simulink model "CRCL"  (R2020b)
settings: Solver=FixedStepDiscrete  StartTime=0.0  StopTime=inf  FixedStep=0.01  RelTol=1e-3  EnableMultiTasking=on
values from neighbouring files (symbols this model uses):
  calibrationDelayTime_s = 2.0    [CRCL_Dictionary.sldd]
  collisionAngleThreshold_deg = 40.0    [CRCL_Dictionary.sldd]
  collisionVarianceThreshold_g2 = 8.0    [CRCL_Dictionary.sldd]
  cpMaxAbortTime_s = 30.0    [CRCL_Dictionary.sldd]
  cpMaxTipOverAngle_deg = 35.0    [CRCL_Dictionary.sldd]
  cpMinEstDistance_m = 50.0    [CRCL_Dictionary.sldd]
  cpMinEstDistanceGnssBased_m = 200.0    [CRCL_Dictionary.sldd]
  cpMinRiddenTime_s = 15.0    [CRCL_Dictionary.sldd]
  cpMinSpeedRiding_kmh = 10.0    [CRCL_Dictionary.sldd]
  cpNumCrankRevolutionThreshold = 5.0    [CRCL_Dictionary.sldd]
  cpSpeedCond2PositiveSpeedChangeTime_s = 5.0    [CRCL_Dictionary.sldd]
  cpSpeedDerivativeThreshold_kmhs = 0.005    [CRCL_Dictionary.sldd]
  cpTimeOutSpeedCond2_s = 15.0    [CRCL_Dictionary.sldd]
  groundHitEnergyThresholdStanding_g2s2 = 0.02    [CRCL_Dictionary.sldd]
  groundHitTipOverAngleThreshold_deg = 40.0    [CRCL_Dictionary.sldd]
  longAccCompForEulerEstFlag = 0.0    [CRCL_Dictionary.sldd]
  minEnergyStrongHit_g2s2 = 0.1    [CRCL_Dictionary.sldd]
  noMotionAccVarianceThresholdSD_g2 = 0.001    [CRCL_Dictionary.sldd]
  ride1minSpeedSlow_kmh = 4.0    [CRCL_Dictionary.sldd]
  ride2minSpeed_kmh = 8.0    [CRCL_Dictionary.sldd]
  rroMaxSpeed_kmh = 5.0    [CRCL_Dictionary.sldd]
  rroMinGyrX_degs = 20.0    [CRCL_Dictionary.sldd]
  rroMonotonyThreshold_degs = -1.0    [CRCL_Dictionary.sldd]
  rroRollIntegrationAngleThreshold_degs = 20.0    [CRCL_Dictionary.sldd]
  rroUniContinuityThreshold_degs = 15.0    [CRCL_Dictionary.sldd]
  scaleFactorVarianceStrongHit = 2.0    [CRCL_Dictionary.sldd]
  sdoMaxAccVarFreeFall_g2 = 0.06    [CRCL_Dictionary.sldd]
  sdoMaxTipOverAngle_deg = 20.0    [CRCL_Dictionary.sldd]
  sdoMinAccVar_g2 = 8.0    [CRCL_Dictionary.sldd]
  sdoMinGyrXYNorm_degs = 720.0    [CRCL_Dictionary.sldd]
  sdoMinGyrXYNormFreeFall_degs = 100.0    [CRCL_Dictionary.sldd]
  sdoMinOrientationChange_deg = 120.0    [CRCL_Dictionary.sldd]
  sdoScaleFactorOrientationChange = 3.0    [CRCL_Dictionary.sldd]
  stepTime_s = 0.01    [CRCL_Dictionary.sldd]
  strongHitSafetyFactor = 2.5    [CRCL_Dictionary.sldd]
  tipOverAccZFiltTreshold_g = 0.7    [CRCL_Dictionary.sldd]
  tipOverAngleThreshold_deg = 50.0    [CRCL_Dictionary.sldd]
  tipOverMinAccZFiltNoseOver_g = 0.3    [CRCL_Dictionary.sldd]
  tipOverRollPitchRelationNoseOver = 1.5    [CRCL_Dictionary.sldd]
undefined symbols (not defined in the file or in its folder): magnitude
libraries: simulink x17
(part 2 of 8)

== system CRCL/Double-Click Button to set current folder ==

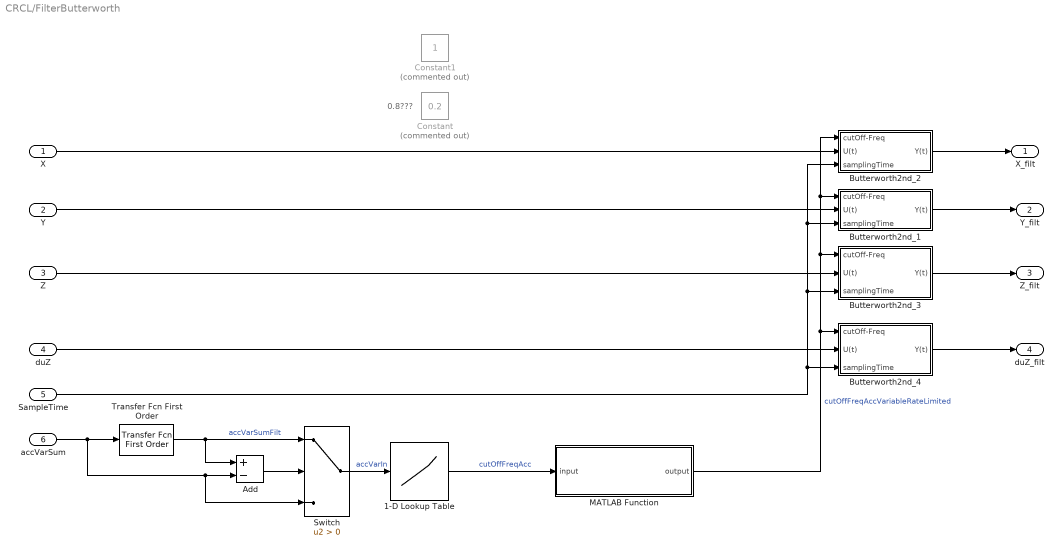
== system CRCL/FilterButterworth ==
  note: 0.8???
  X : Inport
  Y : Inport  Port=2
  Z : Inport  Port=3
  duZ : Inport  Port=4
  SampleTime : Inport  Port=5
  "accVarSum " : Inport  Port=6
  1-D Lookup Table : Lookup_n-D  NumberOfTableDimensions=1  BreakpointsForDimension1=[0 0.0005 0.005 0.01 0.1 50]  Table=[10 10 1 0.5 0.2 0.2]  InternalRulePriority=Speed  RndMeth=Simplest  InputSameDT=on
  Add : Sum  Inputs=+-
  Butterworth2nd_1 : Subsystem
  Butterworth2nd_2 : Subsystem
  Butterworth2nd_3 : Subsystem
  Butterworth2nd_4 : Subsystem
  Constant : Constant  Commented=on  Value=0.2  OutDataTypeStr=single
  Constant1 : Constant  Commented=on
  MATLAB Function : MATLAB Function  TreatAsAtomicUnit=on
  Switch : Switch  Criteria=u2 > Threshold
  Transfer Fcn First Order : simulink/Discrete/Transfer Fcn First Order  PoleZ=0.92  ICPrevOutput=0.0  DoSatur=off
  X_filt : Outport  VectorParamsAs1DForOutWhenUnconnected=off
  Y_filt : Outport  Port=2  VectorParamsAs1DForOutWhenUnconnected=off
  Z_filt : Outport  Port=3  VectorParamsAs1DForOutWhenUnconnected=off
  duZ_filt : Outport  Port=4  VectorParamsAs1DForOutWhenUnconnected=off
  wires:
  Butterworth2nd_2/1(Y(t)) -> X_filt/1
  Butterworth2nd_1/1(Y(t)) -> Y_filt/1
  Butterworth2nd_3/1(Y(t)) -> Z_filt/1
  Z/1 -> Butterworth2nd_3/2(U(t))
  Y/1 -> Butterworth2nd_1/2(U(t))
  X/1 -> Butterworth2nd_2/2(U(t))
  "accVarSum "/1 -> Switch/3, Add/2, Transfer Fcn First Order/1
  Add/1 -> Switch/2
  Transfer Fcn First Order/1 -> Add/1, Switch/1  "accVarSumFilt"
  Switch/1 -> 1-D Lookup Table/1  "accVarIn"
  1-D Lookup Table/1 -> MATLAB Function/1(input)  "cutOffFreqAcc"
  MATLAB Function/1(output) -> Butterworth2nd_4/1(cutOff-Freq), Butterworth2nd_2/1(cutOff-Freq), Butterworth2nd_1/1(cutOff-Freq), Butterworth2nd_3/1(cutOff-Freq)  "cutOffFreqAccVariableRateLimited"
  duZ/1 -> Butterworth2nd_4/2(U(t))
  Butterworth2nd_4/1(Y(t)) -> duZ_filt/1
  SampleTime/1 -> Butterworth2nd_4/3(samplingTime), Butterworth2nd_1/3(samplingTime), Butterworth2nd_2/3(samplingTime), Butterworth2nd_3/3(samplingTime)

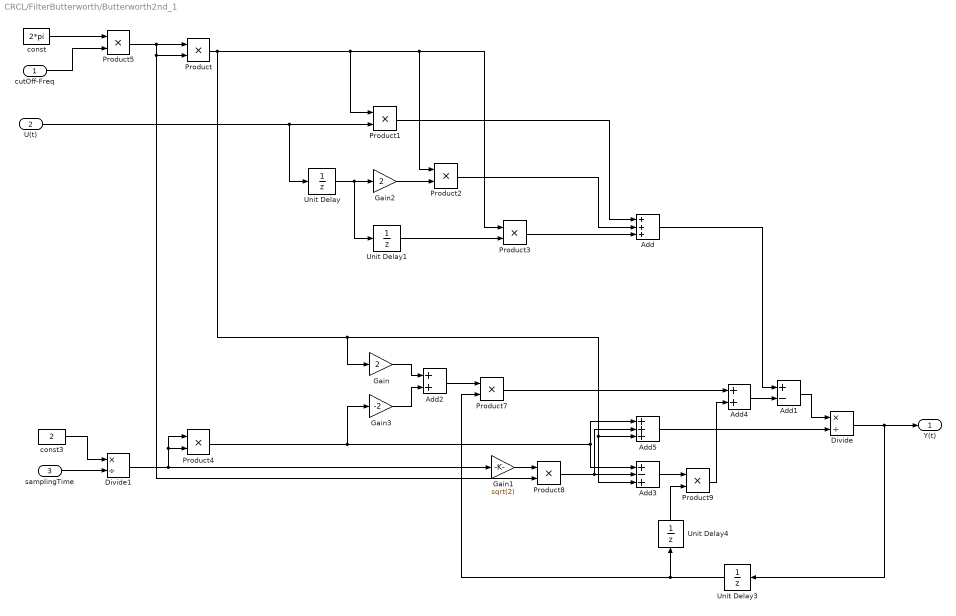
== system CRCL/FilterButterworth/Butterworth2nd_1 ==
  cutOff-Freq : Inport
  U(t) : Inport  Port=2
  samplingTime : Inport  Port=3
  Add : Sum  Inputs=+++
  Add1 : Sum  Inputs=+-
  Add2 : Sum
  Add3 : Sum  Inputs=+-+
  Add4 : Sum
  Add5 : Sum  Inputs=+++
  Divide : Product  Inputs=*/
  Divide1 : Product  Inputs=*/
  Gain : Gain  Gain=2
  Gain1 : Gain  Gain=sqrt(2)
  Gain2 : Gain  Gain=2
  Gain3 : Gain  Gain=-2
  Product{,1..5,7..9} (9 alike) : Product  RndMeth=Zero
  Unit Delay{,1,3..4} (4 alike) : UnitDelay  SampleTime=-1  HasFrameUpgradeWarning=on
  const : Constant  Value=2*pi  OutDataTypeStr=single
  const3 : Constant  Value=2  OutDataTypeStr=single
  Y(t) : Outport  VectorParamsAs1DForOutWhenUnconnected=off
  wires:
  U(t)/1 -> Product1/2, Unit Delay/1
  Product/1 -> Product1/1, Product3/1, Product2/1, Gain/1, Add3/3, Add5/3
  Unit Delay/1 -> Unit Delay1/1, Gain2/1
  Unit Delay1/1 -> Product3/2
  Product1/1 -> Add/1
  Product2/1 -> Add/2
  Product3/1 -> Add/3
  Add/1 -> Add1/1
  Divide/1 -> Unit Delay3/1, Y(t)/1
  Product4/1 -> Add3/1, Add5/1, Gain3/1
  Gain/1 -> Add2/1
  Unit Delay3/1 -> Product7/2, Unit Delay4/1
  Add2/1 -> Product7/1
  Gain1/1 -> Product8/1
  Product8/1 -> Add3/2, Add5/2
  Unit Delay4/1 -> Product9/2
  Add3/1 -> Product9/1
  Product9/1 -> Add4/2
  Product7/1 -> Add4/1
  Add4/1 -> Add1/2
  Add1/1 -> Divide/1
  Add5/1 -> Divide/2
  Gain2/1 -> Product2/2
  Gain3/1 -> Add2/2
  Product5/1 -> Product/1, Product/2, Product8/2
  const/1 -> Product5/1
  cutOff-Freq/1 -> Product5/2
  const3/1 -> Divide1/1
  samplingTime/1 -> Divide1/2
  Divide1/1 -> Gain1/1, Product4/2, Product4/1

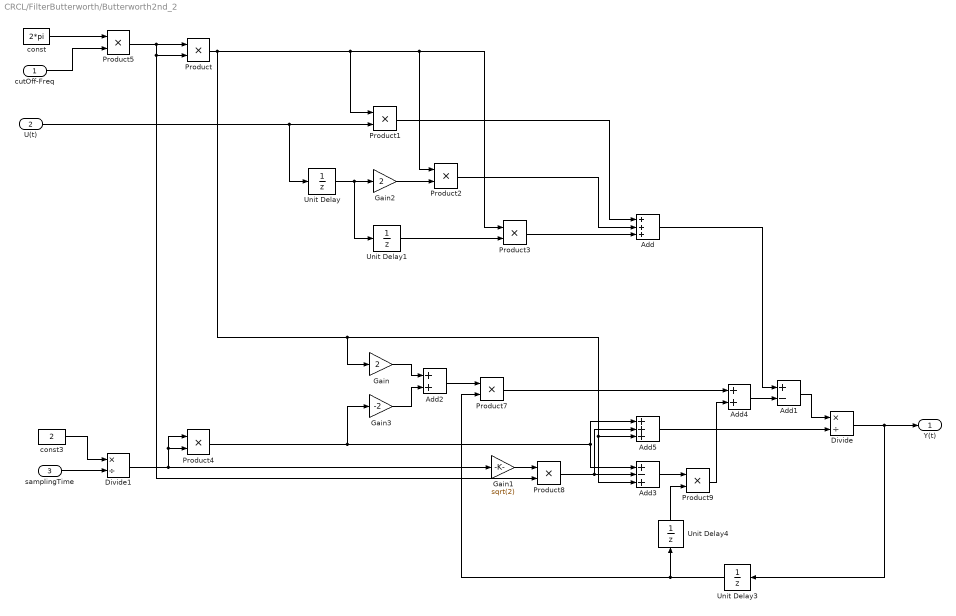
== system CRCL/FilterButterworth/Butterworth2nd_2 ==
  cutOff-Freq : Inport
  U(t) : Inport  Port=2
  samplingTime : Inport  Port=3
  Add : Sum  Inputs=+++
  Add1 : Sum  Inputs=+-
  Add2 : Sum
  Add3 : Sum  Inputs=+-+
  Add4 : Sum
  Add5 : Sum  Inputs=+++
  Divide : Product  Inputs=*/
  Divide1 : Product  Inputs=*/
  Gain : Gain  Gain=2
  Gain1 : Gain  Gain=sqrt(2)
  Gain2 : Gain  Gain=2
  Gain3 : Gain  Gain=-2
  Product{,1..5,7..9} (9 alike) : Product  RndMeth=Zero
  Unit Delay{,1,3..4} (4 alike) : UnitDelay  SampleTime=-1  HasFrameUpgradeWarning=on
  const : Constant  Value=2*pi  OutDataTypeStr=single
  const3 : Constant  Value=2  OutDataTypeStr=single
  Y(t) : Outport  VectorParamsAs1DForOutWhenUnconnected=off
  wires:
  Divide1/1 -> Product4/1, Product4/2, Gain1/1
  samplingTime/1 -> Divide1/2
  const3/1 -> Divide1/1
  cutOff-Freq/1 -> Product5/2
  const/1 -> Product5/1
  Product5/1 -> Product8/2, Product/2, Product/1
  Gain3/1 -> Add2/2
  Gain2/1 -> Product2/2
  Add5/1 -> Divide/2
  Add1/1 -> Divide/1
  Add4/1 -> Add1/2
  Product7/1 -> Add4/1
  Product9/1 -> Add4/2
  Add3/1 -> Product9/1
  Unit Delay4/1 -> Product9/2
  Product8/1 -> Add5/2, Add3/2
  Gain1/1 -> Product8/1
  Add2/1 -> Product7/1
  Unit Delay3/1 -> Unit Delay4/1, Product7/2
  Gain/1 -> Add2/1
  Product4/1 -> Gain3/1, Add5/1, Add3/1
  Divide/1 -> Y(t)/1, Unit Delay3/1
  Add/1 -> Add1/1
  Product3/1 -> Add/3
  Product2/1 -> Add/2
  Product1/1 -> Add/1
  Unit Delay1/1 -> Product3/2
  Unit Delay/1 -> Gain2/1, Unit Delay1/1
  Product/1 -> Add5/3, Add3/3, Gain/1, Product2/1, Product3/1, Product1/1
  U(t)/1 -> Unit Delay/1, Product1/2

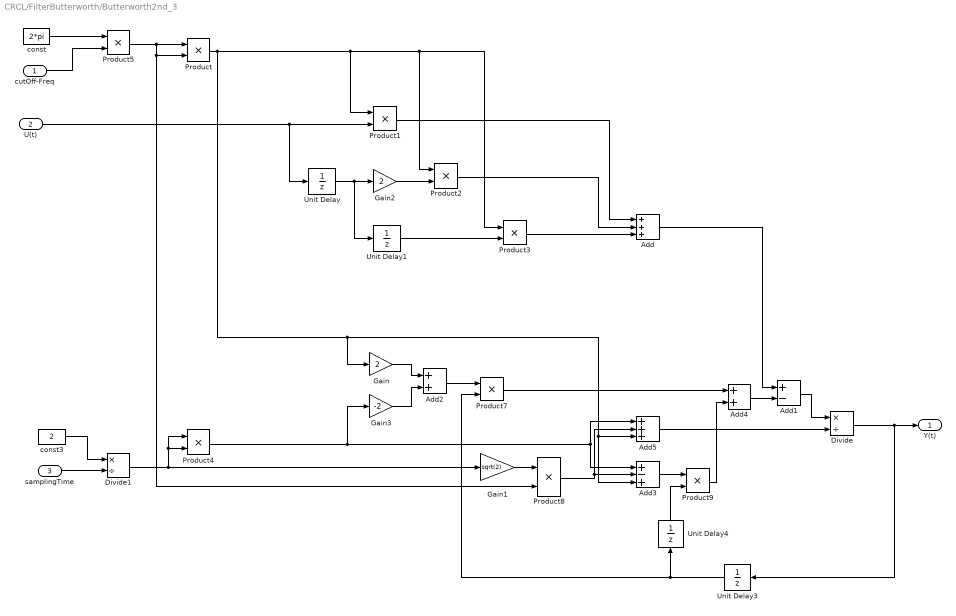
== system CRCL/FilterButterworth/Butterworth2nd_3 ==
  cutOff-Freq : Inport
  U(t) : Inport  Port=2
  samplingTime : Inport  Port=3
  Add : Sum  Inputs=+++
  Add1 : Sum  Inputs=+-
  Add2 : Sum
  Add3 : Sum  Inputs=+-+
  Add4 : Sum
  Add5 : Sum  Inputs=+++
  Divide : Product  Inputs=*/
  Divide1 : Product  Inputs=*/
  Gain : Gain  Gain=2
  Gain1 : Gain  Gain=sqrt(2)
  Gain2 : Gain  Gain=2
  Gain3 : Gain  Gain=-2
  Product{,1..5,7..9} (9 alike) : Product  RndMeth=Zero
  Unit Delay{,1,3..4} (4 alike) : UnitDelay  SampleTime=-1  HasFrameUpgradeWarning=on
  const : Constant  Value=2*pi  OutDataTypeStr=single
  const3 : Constant  Value=2  OutDataTypeStr=single
  Y(t) : Outport  VectorParamsAs1DForOutWhenUnconnected=off
  wires:
  Divide1/1 -> Product4/1, Product4/2, Gain1/1
  samplingTime/1 -> Divide1/2
  const3/1 -> Divide1/1
  cutOff-Freq/1 -> Product5/2
  const/1 -> Product5/1
  Product5/1 -> Product8/2, Product/2, Product/1
  Gain3/1 -> Add2/2
  Gain2/1 -> Product2/2
  Add5/1 -> Divide/2
  Add1/1 -> Divide/1
  Add4/1 -> Add1/2
  Product7/1 -> Add4/1
  Product9/1 -> Add4/2
  Add3/1 -> Product9/1
  Unit Delay4/1 -> Product9/2
  Product8/1 -> Add5/2, Add3/2
  Gain1/1 -> Product8/1
  Add2/1 -> Product7/1
  Unit Delay3/1 -> Unit Delay4/1, Product7/2
  Gain/1 -> Add2/1
  Product4/1 -> Gain3/1, Add5/1, Add3/1
  Add/1 -> Add1/1
  Product3/1 -> Add/3
  Product2/1 -> Add/2
  Product1/1 -> Add/1
  Unit Delay1/1 -> Product3/2
  Unit Delay/1 -> Gain2/1, Unit Delay1/1
  Product/1 -> Add5/3, Add3/3, Gain/1, Product2/1, Product3/1, Product1/1
  U(t)/1 -> Unit Delay/1, Product1/2
  Divide/1 -> Unit Delay3/1, Y(t)/1

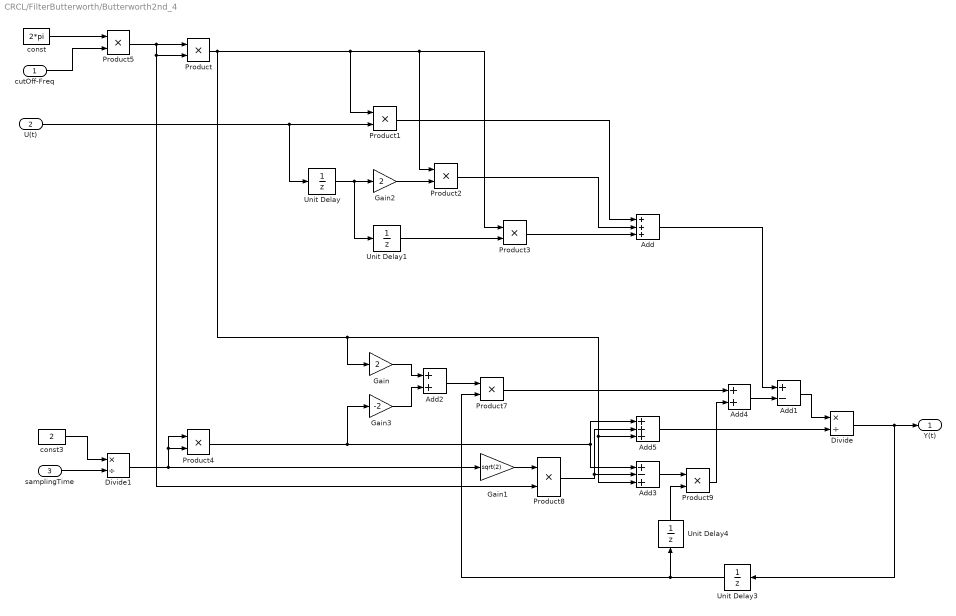
== system CRCL/FilterButterworth/Butterworth2nd_4 ==
  cutOff-Freq : Inport
  U(t) : Inport  Port=2
  samplingTime : Inport  Port=3
  Add : Sum  Inputs=+++
  Add1 : Sum  Inputs=+-
  Add2 : Sum
  Add3 : Sum  Inputs=+-+
  Add4 : Sum
  Add5 : Sum  Inputs=+++
  Divide : Product  Inputs=*/
  Divide1 : Product  Inputs=*/
  Gain : Gain  Gain=2
  Gain1 : Gain  Gain=sqrt(2)
  Gain2 : Gain  Gain=2
  Gain3 : Gain  Gain=-2
  Product{,1..5,7..9} (9 alike) : Product  RndMeth=Zero
  Unit Delay{,1,3..4} (4 alike) : UnitDelay  SampleTime=-1  HasFrameUpgradeWarning=on
  const : Constant  Value=2*pi  OutDataTypeStr=single
  const3 : Constant  Value=2  OutDataTypeStr=single
  Y(t) : Outport  VectorParamsAs1DForOutWhenUnconnected=off
  wires:
  Divide/1 -> Y(t)/1, Unit Delay3/1
  U(t)/1 -> Product1/2, Unit Delay/1
  Product/1 -> Product1/1, Product3/1, Product2/1, Gain/1, Add3/3, Add5/3
  Unit Delay/1 -> Unit Delay1/1, Gain2/1
  Unit Delay1/1 -> Product3/2
  Product1/1 -> Add/1
  Product2/1 -> Add/2
  Product3/1 -> Add/3
  Add/1 -> Add1/1
  Product4/1 -> Add3/1, Add5/1, Gain3/1
  Gain/1 -> Add2/1
  Unit Delay3/1 -> Product7/2, Unit Delay4/1
  Add2/1 -> Product7/1
  Gain1/1 -> Product8/1
  Product8/1 -> Add3/2, Add5/2
  Unit Delay4/1 -> Product9/2
  Add3/1 -> Product9/1
  Product9/1 -> Add4/2
  Product7/1 -> Add4/1
  Add4/1 -> Add1/2
  Add1/1 -> Divide/1
  Add5/1 -> Divide/2
  Gain2/1 -> Product2/2
  Gain3/1 -> Add2/2
  Product5/1 -> Product/1, Product/2, Product8/2
  const/1 -> Product5/1
  cutOff-Freq/1 -> Product5/2
  const3/1 -> Divide1/1
  samplingTime/1 -> Divide1/2
  Divide1/1 -> Gain1/1, Product4/2, Product4/1

== matlab function CRCL/Madgwick IMU MATLAB Function1 ==
  data: AccelerometerX input; AccelerometerY input; AccelerometerZ input; gyrBfX input; gyrBfY input; gyrBfZ input; Beta input; eulerPitch output; eulerRoll output; eulerYaw output; BetaIntern output; SD_fire input; SecondCalibrationDonePeriod input; HD_GroundHit input; HD_CollisionHit input; GyroBiasX output; GyroBiasY output; GyroBiasZ output; SecondCalibrationDone input; curVarSum input
function [eulerPitch, eulerRoll, eulerYaw,...
    BetaIntern, GyroBiasX, GyroBiasY, GyroBiasZ] =  fcn(AccelerometerX, AccelerometerY, AccelerometerZ, ...
    gyrBfX, gyrBfY, gyrBfZ, Beta, SD_fire, SecondCalibrationDonePeriod,...
    HD_GroundHit, HD_CollisionHit, SecondCalibrationDone, curVarSum)

    % calculate centrifugal Acc
    % centrifugalAcc = cross([gyrBfX * pi / 180 ; gyrBfY * pi / 180 ; gyrBfZ * pi / 180],[speed_kmh/3.6; 0; 0]);
    % 
    % centrifualAccX_g = centrifugalAcc(1) / 9.81;
    % centrifualAccY_g = centrifugalAcc(2) / 9.81;
    % centrifualAccZ_g = centrifugalAcc(3) / 9.81;
    % 
    % Accelerometer = [AccelerometerFilteredY + centrifualAccY_g; AccelerometerStrongFilteredX + centrifualAccX_g;...
    %    AccelerometerStrongFilteredZ + centrifualAccZ_g];

%     Accelerometer = [AccelerometerY; AccelerometerX;...
%          AccelerometerZ];
     
    Accelerometer = single([AccelerometerX; AccelerometerY;...
         AccelerometerZ]);
     
     %check Data: if Accelerometer is all zero, Madgwick returns NaN
    if ~any(Accelerometer) 
        Accelerometer = single([0.05; 0.05; 1]);
    end
%     Gyroscope = [gyrBfY; gyrBfX; gyrBfZ];
    Gyroscope = [gyrBfX; gyrBfY; gyrBfZ];

    persistent SamplePeriod Quaternion Step GyroBiasEst Theta gyroBiasFlag

    %% declaration only during first run!

    if isempty(SamplePeriod)
            SamplePeriod = 1/100;
            Quaternion=Start(Accelerometer);
            GyroBiasEst=[0 0 0];
            Theta = 0.000002;
            gyroBiasFlag = 0;
    end

    if SD_fire && (HD_GroundHit == 1 || HD_CollisionHit == 1)
        BetaIntern =  200 * Beta;
    elseif SD_fire == 1 || SecondCalibrationDonePeriod == 1  
        BetaIntern =  100 * Beta;
%     elseif SecondCalibrationDone == 1 && curVarSum <= 0.015
%         BetaIntern =  25 * Beta;
    else
        BetaIntern =  Beta;
    end
    
    q =  Quaternion; % short name local variable for readability, Jan: Quaternion represents Orientation
    Gyroscope = Gyroscope *(pi/180);

    %Centrifugal_acc = cross(Gyroscope, [Speed 0  0])/9.81;      %speed in m/s
    %Accelerometer =  Accelerometer - Centrifugal_acc';
    
	% Gradient decent algorithm corrective Step
            F = [2*(q(2)*q(4) - q(1)*q(3)) - Accelerometer(1)
                2*(q(1)*q(2) + q(3)*q(4))  - Accelerometer(2)
                2*(0.5 - q(2)^2 - q(3)^2)  - Accelerometer(3)];
            J = [-2*q(3),	2*q(4),    -2*q(1),	2*q(2)
                2*q(2),     2*q(1),     2*q(4),	2*q(3)
                0,         -4*q(2),    -4*q(3),	0    ];
	Step = (J'*F);
	Step = Step / norm(Step);	% normalise Step magnitude
    
    if gyroBiasFlag == 1 || SecondCalibrationDonePeriod == 1
        gyroBiasFlag = 1;
        So = 2 * quaternProd(quaternConj(q), (Step / norm(Step))');
        GyroBiasEst = GyroBiasEst + Theta .* So(2:end); 
    end

    
% 	gravity = [2*(q(2)*q(4) - q(1)*q(3))
% 			2*(q(1)*q(2) + q(3)*q(4))
% 			2*(0.5 - q(2)^2 - q(3)^2)];

    % 		So = 2 * quaternProd(quaternConj(q), (Step / norm(Step))');
    % 		qDot = 0.5 * quaternProd(q, [0 Gyroscope(1)- GyroBias(1) Gyroscope(2)- GyroBias(2) Gyroscope(3)- GyroBias(3)]) - BetaIntern * Step';
    qDot = 0.5 * quaternProd(q, [0 Gyroscope(1)-GyroBiasEst(1) Gyroscope(2)-GyroBiasEst(2) Gyroscope(3)-GyroBiasEst(3)]) - BetaIntern * Step';

    % Integrate to yield quaternion
    q = q + qDot *  SamplePeriod;
    Quaternion = q / norm(q); % normalise quaternion
    euler = quatern2euler(quaternConj(Quaternion)) * (180/pi);	% use conjugate for sensor frame relative to Earth and convert to degrees.
    %euler = unwrap(euler,180);
    eulerRoll = euler(1);
    eulerPitch = euler(2);
    eulerYaw = euler(3);
    
    GyroBiasX = GyroBiasEst(1)*180/pi;
    GyroBiasY = GyroBiasEst(2)*180/pi;
    GyroBiasZ = GyroBiasEst(3)*180/pi;
    
end

 function [Quat] = Start(Accelerometer)
    stepper=single([1 1 1 1]');
    Quat=single([1 0 0 0]);
    while norm(stepper) >= 1e-2
        [Quat, stepper]= Update(Accelerometer, single([0 0 0]) , Quat(1,1:4),stepper(1:4));
    end            
 end

function [Quat, stepper] = Update(Accelerometer, Gyroscope, Quat, stepper)

persistent SamplePeriod Quaternion GyroBias Theta Step
%% declaration only during first run!

if isempty(SamplePeriod)
        SamplePeriod = single(1/100);
        Quaternion = single([1 0 0 0]);     % output quaternion describing the Earth relative to the sensor
%         GyroBias = [-1 1 0]*pi/180;
        GyroBias = single([0 0 0]);        
        Theta = single(0.00001);
        Step = single([0 0 0 0]');
     
               
end
% 	euler=zeros(1,3);
	q =  Quaternion; % short name local variable for readability, Jan: Quaternion represents Orientation
           
	BetaIntern = 0.9;
	
	Gyroscope=Gyroscope* (pi/180);
	
	% Normalise accelerometer measurement
	Accelerometer = Accelerometer / norm(Accelerometer);	% normalise magnitude
	% Gradient decent algorithm corrective Step
            F = [2*(q(2)*q(4) - q(1)*q(3)) - Accelerometer(1)
                2*(q(1)*q(2) + q(3)*q(4))  - Accelerometer(2)
                2*(0.5 - q(2)^2 - q(3)^2)  - Accelerometer(3)];
            J = [-2*q(3),	2*q(4),    -2*q(1),	2*q(2)
                2*q(2),     2*q(1),     2*q(4),	2*q(3)
                0,         -4*q(2),    -4*q(3),	0    ];
	Step = (J'*F);
	stepper = Step;
	Step = Step / norm(Step);	% normalise Step magnitude
	
	% Compute rate of change of quaternion
	
	gravity = [2*(q(2)*q(4) - q(1)*q(3))
			2*(q(1)*q(2) + q(3)*q(4))
			2*(0.5 - q(2)^2 - q(3)^2)];

		So = 2 * quaternProd(quaternConj(q), (Step / norm(Step))');
		%GyroBias =  GyroBias +  Theta .* So(2:end);  
		%qDot = 0.5 * quaternProd(q, [0 Gyroscope(1)- GyroBias(1) Gyroscope(2)- GyroBias(2) Gyroscope(3)- GyroBias(3)]) -  Beta * Step';
		qDot = 0.5 * quaternProd(q, [0 Gyroscope(1)- GyroBias(1) Gyroscope(2)- GyroBias(2) Gyroscope(3)- GyroBias(3)]) - BetaIntern * Step';
	
	% Integrate to yield quaternion
	q = q + qDot *  SamplePeriod;
	Quaternion = q / norm(q); % normalise quaternion
	Quat=Quaternion;
%              euler = quatern2euler(quaternConj(Quaternion)) * (180/pi);	% use conjugate for sensor frame relative to Earth and convert to degrees.
%              euler = unwrap(euler,180);

end

function euler = quatern2euler(q)
%QUATERN2EULER Converts a quaternion orientation to ZYX Euler angles
%
%   q = quatern2euler(q)
%
%   Converts a quaternion orientation to ZYX Euler angles where phi is a
%   rotation around X, theta around Y and psi around Z.
%
%   For more information see:
%   http://www.x-io.co.uk/node/8#quaternions
%
%	Date          Author          Notes
%	27/09/2011    SOH Madgwick    Initial release
% R = zeros(3,3,1);
%     R(1,1,:) = 2.*q(:,1).^2-1+2.*q(:,2).^2;
%     R(2,1,:) = 2.*(q(:,2).*q(:,3)-q(:,1).*q(:,4));
%     R(3,1,:) = 2.*(q(:,2).*q(:,4)+q(:,1).*q(:,3));
%     R(3,2,:) = 2.*(q(:,3).*q(:,4)-q(:,1).*q(:,2));
%     R(3,3,:) = 2.*q(:,1).^2-1+2.*q(:,4).^2;
% 
%     phi = atan2(R(3,2,:), R(3,3,:) );
%     theta = -atan(R(3,1,:) ./ sqrt(1-R(3,1,:).^2) );
%     psi = atan2(R(2,1,:), R(1,1,:) );
% 
%     euler = [phi(1,:)' theta(1,:)' psi(1,:)'];
    
    R = zeros(3,3);
    R(1,1) = 2.*q(1).^2-1+2.*q(2).^2;
    R(2,1) = 2.*(q(2).*q(3)-q(1).*q(4));
    R(3,1) = 2.*(q(2).*q(4)+q(1).*q(3));
    R(3,2) = 2.*(q(3).*q(4)-q(1).*q(2));
    R(3,3) = 2.*q(1).^2-1+2.*q(4).^2;

    phi = atan2(R(3,2), R(3,3));
    theta = -atan(R(3,1) ./ sqrt(1-R(3,1).^2) );
    psi = atan2(R(2,1), R(1,1) );

    euler = [phi theta psi];
end

function qConj = quaternConj(q)
%QUATERN2ROTMAT Converts a quaternion to its conjugate
%
%   qConj = quaternConj(q)
%
%   Converts a quaternion to its conjugate.
%
%   For more information see:
%   http://www.x-io.co.uk/node/8#quaternions
%
%	Date          Author          Notes
%	27/09/2011    SOH Madgwick    Initial release

    qConj = [q(:,1) -q(:,2) -q(:,3) -q(:,4)];
end


function ab = quaternProd(a, b)
%QUATERNPROD Calculates the quaternion product
%
%   ab = quaternProd(a, b)
%
%   Calculates the quaternion product of quaternion a and b.
%
%   For more information see:
%   http://www.x-io.co.uk/node/8#quaternions
%
%	Date          Author          Notes
%	27/09/2011    SOH Madgwick    Initial release
%     ab = zeros(1,4);
%     ab(:,1) = a(:,1).*b(:,1)-a(:,2).*b(:,2)-a(:,3).*b(:,3)-a(:,4).*b(:,4);
%     ab(:,2) = a(:,1).*b(:,2)+a(:,2).*b(:,1)+a(:,3).*b(:,4)-a(:,4).*b(:,3);
%     ab(:,3) = a(:,1).*b(:,3)-a(:,2).*b(:,4)+a(:,3).*b(:,1)+a(:,4).*b(:,2);
%     ab(:,4) = a(:,1).*b(:,4)+a(:,2).*b(:,3)-a(:,3).*b(:,2)+a(:,4).*b(:,1);
%     
        ab = zeros(1,4);
    ab(1,1) = a(1,1).*b(1,1)-a(1,2).*b(1,2)-a(1,3).*b(1,3)-a(1,4).*b(1,4);
    ab(1,2) = a(1,1).*b(1,2)+a(1,2).*b(1,1)+a(1,3).*b(1,4)-a(1,4).*b(1,3);
    ab(1,3) = a(1,1).*b(1,3)-a(1,2).*b(1,4)+a(1,3).*b(1,1)+a(1,4).*b(1,2);
    ab(1,4) = a(1,1).*b(1,4)+a(1,2).*b(1,3)-a(1,3).*b(1,2)+a(1,4).*b(1,1);
end

function q = angle2quatern( r1, r2, r3 )


angles = [r1 r2 r3];

cang = cos( angles/2 );
sang = sin( angles/2 );

        q = [ cang(1).*cang(2).*cang(3) + sang(1).*sang(2).*sang(3), ...
            cang(1).*cang(2).*sang(3) - sang(1).*sang(2).*cang(3), ...
            cang(1).*sang(2).*cang(3) + sang(1).*cang(2).*sang(3), ...
            sang(1).*cang(2).*cang(3) - cang(1).*sang(2).*sang(3)];
end

== stateflow chart CRCL/StandDetection_SD ==
  state StandDetectionWithoutSpeed [parallel]
    settings: executionOrder=1
    state Init
      en:
      SD_StandFire = int16(1);
    note: only IMU based, no Speed
    state waitState
    state CheckVarianceStillRiding
    state Riding
    state Standing
    state CheckVarianceStillStanding
    (default) -> Init
    Init -> waitState : [after(0.5,sec)]
    waitState -> Standing [order 2] : [SD_curVarSum <= SD_varianceThreshold_g2 && ...
        | SD_curGyrMotion == 0]
        | {
        | SD_StandFire = int16(1);
        | }
    waitState -> Riding [order 1] : [SD_curVarSum > SD_varianceThreshold_g2 || ...
        | SD_curGyrMotion == 1]
        | {
        | SD_StandFire = int16(0);
        | }
    Riding -> CheckVarianceStillRiding : [SD_curVarSum <= SD_varianceThreshold_g2 && ...
        | SD_curGyrMotion == 0]
    CheckVarianceStillRiding -> Standing [order 2] : [after(0.25,sec)]
        | {
        | SD_StandFire = int16(1);
        | }
    CheckVarianceStillRiding -> Riding [order 1] : [SD_curVarSum > SD_varianceThreshold_g2 || ...
        | SD_curGyrMotion == 1]
    CheckVarianceStillStanding -> Riding [order 1] : [after(0.02,sec)]
        | {
        | SD_StandFire = int16(0);
        | }
    Standing -> CheckVarianceStillStanding : [SD_curVarSum > SD_varianceThreshold_g2 || ...
        | SD_curGyrMotion == 1]
    CheckVarianceStillStanding -> Standing [order 2] : [SD_curVarSum <= SD_varianceThreshold_g2 && ...
        | SD_curGyrMotion == 0]
  data: SD_curGyrMotion input; SD_curVarSum input; SD_StandFire output; SD_varianceThreshold_g2 input

== stateflow chart CRCL/TipOver ==
  state TipOverSchneeV3
    state Init_
      en:
      %TO_TIPOVER_THRESHOLD = 70; % in degree
      %TO_TIPOVER_THRESHOLD_ROLL = single(55); % 60, in degree
      %TO_TIPOVER_THRESHOLD = 55; % in degree
      %TO_TIPOVER_THRESHOLD_PITCH = single(50); % in degree
      TO_Latchtime = single(2);
      TO_fire = uint8(0);
      TO_curAngle = single(0);
    state WaitForCalibration
      en:
      TO_fire = uint8(0);
    state NoCalibrationButRollOver [commented out]
      en:
      TO_fire = uint8(3);
    state CheckOrientation
      en:
      TO_fire = uint8(0);
      du:
      TO_curAngle = single(TO_curRoll_deg);
    state WaitState
      %waitForLatchtime
      entry:
      TO_curAngle = single(TO_curRoll_deg);
      du:
      TO_curAngle = single(TO_curRoll_deg);
    state waitForAccZfilter1
    note: REMOVED DIVISION BY ZERO!!!
    state waitForAccZfilter
      en:
      TO_noseoverTime_s = TO_noseoverTime_s + timestep;
      du:
      TO_noseoverTime_s = TO_noseoverTime_s + timestep;
    state waitForLatchtime
    state waitForRideFireInternCF
      %RD_fireIntern needs
      %another step
      %in this case for resetting
    (default) -> Init_
    Init_ -> WaitForCalibration
    WaitForCalibration -> NoCalibrationButRollOver [commented out] : [abs(TO_curAccFiltYg)>= 0.6 && TO_systemConfig == 2]
    NoCalibrationButRollOver -> WaitForCalibration [commented out] : [abs(TO_curAccFiltYg) <= 0.4]
    WaitForCalibration -> CheckOrientation : [TO_CalibrationStatus == 1]
    waitForAccZfilter1 -> WaitState [order 2] : [TO_curAccTipOverAngle >= TO_angleThresholdForTO1_deg && TO_cobiHubSetup ~= 2]
        | {
        | TO_fire = uint8(2);
        | }
    WaitState -> WaitState [order 1] : [TO_curTipOverAngle_deg >= TO_angleThresholdForTO1_deg]
    CheckOrientation -> waitForAccZfilter1 [order 2] : [TO_curTipOverAngle_deg >= TO_angleThresholdForTO1_deg]
        | {
        | TO_fire = uint8(1);
        | }
    waitForAccZfilter1 -> CheckOrientation [order 3] : [after(3,sec)]
        | {
        | TO_curAngle = single(0);
        | }
    waitForAccZfilter1 -> (junction 162) [order 1] : %confirmation for smartphoneHub usecase,
        | %use du acc signals, too
        | [TO_cobiHubSetup == 2]
    (junction 162) -> WaitState [order 1] : [TO_curDuAccZFiltG <= TO_accZFiltThreshold_g && ...
        | TO_hubConnection == 1]
        | {
        | TO_fire = uint8(2);
        | }
    (junction 162) -> WaitState [order 2] : %no HubConnection
        | [TO_hubConnection == 0 && ...
        | TO_curAccTipOverAngle >= TO_angleThresholdForTO1_deg]
        | {
        | TO_fire = uint8(2);
        | }
    WaitState -> CheckOrientation [order 2] : [after(TO_Latchtime,sec)]
        | {
        | TO_curAngle = single(0);
        | }
    waitForLatchtime -> waitForLatchtime [order 1] : [TO_curTipOverAngle_deg >= TO_angleThresholdForTO1_deg]
    waitForAccZfilter -> waitForLatchtime [order 3] : [TO_curAccTipOverAngle >= TO_angleThresholdForTO1_deg && TO_cobiHubSetup ~= 2]
        | %abs(TO_curRoll_deg) >= TO_TIPOVER_THRESHOLD_ROLL]
        | %Bike has to lay flat after noseover
        | % -->  stoppie and  assembly stand scenarios should not fire TO = 2!
        | {
        | TO_fire = uint8(3);
        | }
    CheckOrientation -> waitForAccZfilter [order 1] : % Noseover ->Pitch
        | %[TO_curPitch_deg >= TO_angleThresholdForTO1_deg
        | [TO_curTipOverAngle_deg >= TO_angleThresholdForTO1_deg && ...
        | abs(TO_curAccFiltZg) >= TO_minAccZFiltNoseOver_g && ... %this indicates that bicycle was upright befor!
        | TO_curPitch_deg/abs(TO_curRoll_deg) >= TO_rollPitchRelationNoseOver] %accZ Condition might be bad for noseOvers during jumps
        | {
        | TO_fire = uint8(1);
        | TO_noseoverTime_s = single(0);
        | }
    waitForAccZfilter -> waitForAccZfilter [order 5] : [TO_curTipOverAngle_deg >= TO_angleThresholdForTO1_deg]
    waitForAccZfilter -> waitForRideFireInternCF [order 1] : [TO_noseoverTime_s >= 6]
        | {
        | TO_curAngle = single(0);
        | TO_fire = uint8(0);
        | }
    waitForRideFireInternCF -> CheckOrientation
    waitForAccZfilter -> waitForLatchtime [order 4] : %confirmation for smartphoneHub usecase, use du acc signals, too
        | [TO_cobiHubSetup == 2 && TO_curDuAccZFiltG <= TO_accZFiltThreshold_g]
        | {
        | TO_fire = uint8(3);
        | }
    waitForAccZfilter -> CheckOrientation [order 2] : [after(3,sec)]
        | {
        | TO_curAngle = single(0);
        | }
    waitForLatchtime -> CheckOrientation [order 2] : [after(TO_Latchtime,sec)]
        | {
        | TO_curAngle = single(0);
        | }
  data: TO_curAccFiltZg input; TO_fire output uint8; TO_Latchtime local; TO_curAngle output; timestep input; TO_curRoll_deg input; TO_curPitch_deg input; TO_curTipOverAngle_deg input; TO_noseoverTime_s local; TO_CalibrationStatus input; TO_curAccTipOverAngle input; TO_cobiHubSetup input; TO_curDuAccZFiltG input; TO_angleThresholdForTO1_deg input; TO_accZFiltThreshold_g input; TO_minAccZFiltNoseOver_g input; TO_rollPitchRelationNoseOver input; TO_hubConnection input

== matlab function CRCL/MATLAB Function2 ==
  data: gyrX input; gyrY input; gyrZ input; accX input; accY input; accZ input; varAccX output; varAccY output; varAccZ output; varGyrX output; varGyrY output; varGyrZ output; impulseX output; impulseY output; impulseZ output; stepTime_s input; extremaAccValY output; roll_deg input; pitch_deg input; impulseShortTermX output; impulseShortTermY output
function [varAccX, varAccY, varAccZ, ...
    varGyrX, varGyrY, varGyrZ, ...
    impulseX, impulseY, impulseZ, ...
    extremaAccValY, ...
    impulseShortTermX, impulseShortTermY] = ...
    varPastNumSamples(gyrX, gyrY, gyrZ, ...
    accX, accY, accZ, stepTime_s, roll_deg, pitch_deg)

persistent ringBufAccX ringBufAccY ringBufAccZ i ringBufXgComp ringBufYgComp ...
    ringBufZgComp NumSamplesLongtermIntern NumSamplesShortTermIntern ...
    ringBufGyrX ringBufGyrY ringBufGyrZ
        
%% declaration only during first run!
gCompensation = 1;

if isempty(i)  
        NumSamplesLongtermIntern = int16(7);
        NumSamplesShortTermIntern = int16(5);
        
%% for crash feature evaluation --> different buffer sizes...
%         ringBufX = single(zeros(NumSamplesLongtermIntern,1));
%         ringBufY = single(zeros(NumSamplesLongtermIntern,1));
%         ringBufZ = single(zeros(NumSamplesLongtermIntern,1));
%         ringBufYgComp = single(zeros(NumSamplesLongtermIntern,1));
%         ringBufXgComp = single(zeros(NumSamplesLongtermIntern,1));
%         ringBufZgComp = single(zeros(NumSamplesLongtermIntern,1));
%         ringBufmaxImpulseZ = single(zeros(NumlatchedImpulseZ,1));
%%
        ringBufAccX = single(zeros(7,1));   % variable from NumSamplesLongtermIntern
        ringBufAccY = single(zeros(7,1));   % variable from NumSamplesLongtermIntern
        ringBufAccZ = single(zeros(7,1));   % variable from NumSamplesLongtermIntern
        ringBufXgComp = single(zeros(7,1)); % variable from NumSamplesLongtermIntern
        ringBufYgComp = single(zeros(7,1)); % variable from NumSamplesLongtermIntern
        ringBufZgComp = single(zeros(7,1)); % variable from NumSamplesLongtermIntern
        ringBufGyrX = single(zeros(7,1));   % variable from NumSamplesLongtermIntern
        ringBufGyrY = single(zeros(7,1));   % variable from NumSamplesLongtermIntern
        ringBufGyrZ = single(zeros(7,1));   % variable from NumSamplesLongtermIntern
        
        i = int16(1); 
end

ringBufAccX(i) = accX;
ringBufAccY(i) = accY;
ringBufAccZ(i) = accZ;

ringBufGyrX(i) = gyrX;
ringBufGyrY(i) = gyrY;
ringBufGyrZ(i) = gyrZ;

ringBufXgComp(i) = accX + sind(pitch_deg);
ringBufYgComp(i) = accY - sind(roll_deg);
ringBufZgComp(i) = accZ - cosd(pitch_deg);



varAccX = single(var(ringBufAccX, 0));
varAccY = single(var(ringBufAccY, 0));
varAccZ = single(var(ringBufAccZ, 0));


varGyrX = single(var(ringBufGyrX, 0));
varGyrY = single(var(ringBufGyrY, 0));
varGyrZ = single(var(ringBufGyrZ, 0));



%% for crash feature evaluation --> different buffer sizes...
% indicesMutedLatchedImpulseZ = b-4:b;
% 
% for a=1:length(indicesMutedLatchedImpulseZ)
%     if indicesMutedLatchedImpulseZ(a) <= 0
%         indicesMutedLatchedImpulseZ(a) = indicesMutedLatchedImpulseZ(a)+ NumlatchedImpulseZ;
%     end
% end


%indicesShortTerm = i-(NumSamplesShortTermIntern-1):i;

% for a=1:length(indicesShortTerm)
%     if indicesShortTerm(a) <= 0
%         indicesShortTerm(a) = indicesShortTerm(a)+ NumSamplesLongtermIntern;
%     end
% end

%%

indicesShortTerm = int16(zeros(5,1));   % variable from NumSamplesShortTermIntern
indicesShortTerm(1) = i-4;
indicesShortTerm(2) = i-3;
indicesShortTerm(3) = i-2;
indicesShortTerm(4) = i-1;
indicesShortTerm(5) = i;

for a=1:5
    if indicesShortTerm(a) <= 0
        indicesShortTerm(a) = indicesShortTerm(a)+ NumSamplesLongtermIntern;
    end
end


if  gCompensation == 1
    impulseX = sum(ringBufXgComp.*stepTime_s);
    impulseY = sum(ringBufYgComp.*stepTime_s);
    impulseZ = sum(ringBufZgComp.*stepTime_s);
    impulseShortTermX = sum(ringBufXgComp(indicesShortTerm).*stepTime_s);
    impulseShortTermY = sum(ringBufYgComp(indicesShortTerm).*stepTime_s);
    %impulseShortTermZ = sum(ringBufAccZ(indicesShortTerm).*stepTime_s);
else
    impulseX = sum(ringBufAccX.*stepTime_s);
    impulseY = sum(ringBufAccY.*stepTime_s);
    impulseZ = sum(ringBufAccZ.*stepTime_s);
    impulseShortTermX = sum(ringBufAccX(indicesShortTerm).*stepTime_s);
    impulseShortTermY = sum(ringBufAccY(indicesShortTerm).*stepTime_s);
    %impulseShortTermZ = sum(ringBufAccZ(indicesShortTerm).*stepTime_s);
end

[extremaAccValY, extremaIndY] = max(abs(ringBufAccY));
% if sign(ringBufAccY(extremaIndY)) == 1
%    %extremaAccValY = extremaAccValY;
% else
%     extremaAccValY = extremaAccValY * -1;
% end
if ringBufAccY(extremaIndY) < 0
    extremaAccValY = extremaAccValY * -1;
end

i = i + 1;
if i > NumSamplesLongtermIntern
    i = int16(1);
end

end
